simulink library "thc"  (R2021b)
settings: Solver=VariableStepAuto  StartTime=0.0  StopTime=10.0  RelTol=1e-3
undefined symbols (not defined in the file): ATHC_APTCQA_X_C, ATHC_APTCQB_X_C, ATHC_dAy_X_C, ATHC_Qeq_X_kmh, ATHC_VbaseC_X_C, ATHC_VbaseC_Y_W, ATHC_VbaseD_X_C, ATHC_VbaseH_X_C, FALSE, KTHC_ACMaxMinT_sec, KTHC_aDeice_K, KTHC_AGSDefLv_K, KTHC_AGSLv1_K, KTHC_AGSLv2_K, KTHC_AGSLv3_K, KTHC_AGSLv4_K, KTHC_AGSLv5_K, KTHC_AirIntUpdateT_sec, KTHC_APTCOneZoneMax_W, KTHC_APTCPeriod_cnt, KTHC_APTCPWMEN_flg, KTHC_APTCQMaxC_W, KTHC_APTCQminC_W, KTHC_APTCQminD_W, KTHC_APTCQminRe1_W, KTHC_APTCQminRe_W, KTHC_APTCQoffT_cnt, KTHC_APTCQonT_cnt, KTHC_APTCRiLeMaxDff_W, KTHC_APTCRiLeMinDff_W, KTHC_BatCoolT_cnt, KTHC_BatInTempDef_C, KTHC_bDeice_K, KTHC_CompMaxDeice_rpm, KTHC_CompMinDeice_rpm, KTHC_CompSotxvOp_K, KTHC_CompSotxvOpLow_rpm, KTHC_CompSpdmax_rpm, KTHC_CompSpdmaxBC1_rpm, KTHC_CompSpdmaxBC_rpm, KTHC_CompSpdmid1_rpm, KTHC_CompSpdmid2_rpm, KTHC_CompSpdmid3_rpm, KTHC_CompSpdmid_rpm, KTHC_CompSpdmin_rpm, KTHC_DAPTCQ1_W, KTHC_DAPTCQ2_W, KTHC_DAPTCQ3_W, KTHC_DcChSetTemp_C, KTHC_DehumidityEN_flg, KTHC_DeiceCycTime_K, KTHC_DriveLevelWPTCBAH1_W, KTHC_DriveLevelWPTCBAH2_W, KTHC_DriveLevelWPTCBAH3_W, KTHC_DriveLevelWPTCBAH4_W, KTHC_DriverSeatPos_flg, KTHC_DriveT1MinBAH_C, KTHC_DriveT2MaxBAH_C, KTHC_DriveT2MinBAH_C, KTHC_DriveT3MaxBAH_C ... (+379)
libraries: simulink x489
(part 1 of 17)
settings Model: Creator=FVT20341  LastModifiedBy=FVT22063

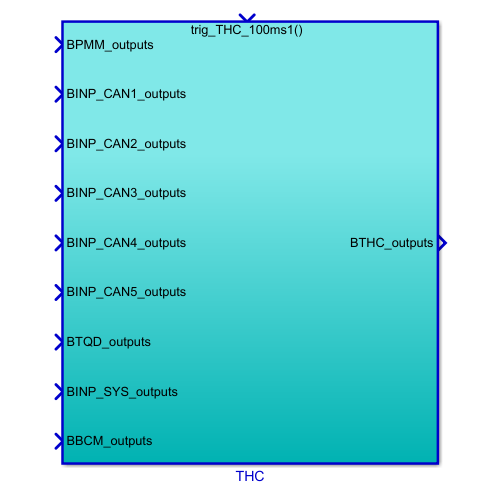
[thumbnail: Simulink's stored preview of the top-level diagram]
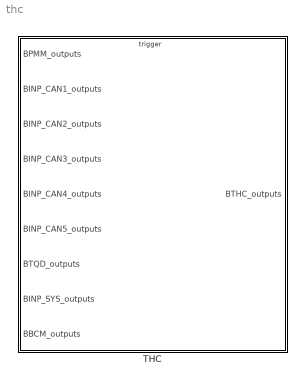
== system thc ==
  THC : Subsystem  TreatAsAtomicUnit=on
      settings: RTWSystemCode=Nonreusable function  RTWFcnNameOpts=Use subsystem name  RTWFileNameOpts=Use subsystem name

== system thc/THC ==
  BPMM_outputs : Inport  OutDataTypeStr=Bus: BPMM_outputs
  BINP_CAN1_outputs : Inport  Port=2  OutDataTypeStr=Bus: BINP_CAN1_outputs
  BINP_CAN2_outputs : Inport  Port=3  OutDataTypeStr=Bus: BINP_CAN2_outputs
  BINP_CAN3_outputs : Inport  Port=4  OutDataTypeStr=Bus: BINP_CAN3_outputs
  BINP_CAN4_outputs : Inport  Port=5  OutDataTypeStr=Bus: BINP_CAN4_outputs
  BINP_CAN5_outputs : Inport  Port=6  OutDataTypeStr=Bus: BINP_CAN5_outputs
  BTQD_outputs : Inport  Port=7  OutDataTypeStr=Bus: BTQD_outputs
  BINP_SYS_outputs : Inport  Port=8  OutDataTypeStr=Bus: BINP_SYS_outputs
  BBCM_outputs : Inport  Port=9  OutDataTypeStr=Bus: BBCM_outputs
  trig_THC_100ms1 : TriggerPort  TriggerType=function-call  VariantControl=(inherit)
  Bus Creator : BusCreator  Inputs=202  OutDataTypeStr=Bus: BTHC_outputs  NonVirtualBus=on
  Bus Selector : BusSelector  OutputSignals=VINP_FlashACModeMem_enum,VINP_FlashFace_enum,VINP_FlashFoot_enum,VINP_FlashFrost_enum,VINP_FlashFaceM_enum,VINP_FlashFootM_enum,VINP_FlashCCUSyncSts_enum,VINP_FlashACForceOFF_flg,VINP_FlashsigRecircSt_enum,VINP_FlashRecAutoFlg_enum,VINP_FlashAirIntenZone1M_enum,VINP_Flashfdefog_enum,VINP_FlashsigSetTempZon1St_C,VINP_FlashsigSetTempZon2StM_C,VINP_FlashAirIntZ3Sta_enum,VINP_FlashREVentModeSta_enum,VINP_FlashLEVentModeSta_enum,VINP_FlashLEVentZSta_enum,VINP_FlashCLEVentZSta_enum,VINP_FlashREVentZSta_enum,VINP_FlashCREVentZSta_enum,VINP_FlashLVentEN_enum,VINP_FlashLEVentYSta_enum,VINP_FlashCLVentEN_enum,VINP_FlashCLEVentYSta_enum,VINP_FlashRVentEN_enum,VINP_FlashREVentYSta_enum,VINP_FlashCRVentEN_enum,VINP_FlashCREVentYSta_enum,VINP_FlashFGSAirIntSta_enum,VINP_FlashFGSChSta_enum,VINP_FlashFGSIONSWSta_enum,VINP_FlashAirIntenZone1MSet2_enum,VINP_FlashAirIntenZone1MSet3_enum,VINP_FlashAirIntenZone1MSet4_enum,VINP_FlashAirIntenZone1MSet5_enum,VINP_FlashAirIntenZone1MSet7_enum,VINP_FlashAirIntenZone3MSet2_enum,VINP_FlashAirIntenZone3MSet3_enum,VINP_FlashAirIntenZone3MSet4_enum,VINP_FlashAirIntenZone3MSet5_enum,VINP_FlashAirIntenZone3MSet7_enum,VINP_FlashFGSChStaSet457_enum,VINP_FlashFGSAirIntStaSet457_enum,VINP_FlashLEVentModeStaSet457_enum,VINP_FlashREVentModeStaSet457_enum,VINP_FlashLEVentZStaSet2_enum,VINP_FlashLEVentZStaSet3_enum,VINP_FlashLEVentZStaSet4_enum,VINP_FlashLEVentZStaSet5_enum,VINP_FlashLEVentZStaSet7_enum,VINP_FlashCLEVentZStaSet2_enum,VINP_FlashCLEVentZStaSet3_enum,VINP_FlashCLEVentZStaSet4_enum,VINP_FlashCLEVentZStaSet5_enum,VINP_FlashCLEVentZStaSet7_enum,VINP_FlashREVentZStaSet2_enum,VINP_FlashREVentZStaSet3_enum,VINP_FlashREVentZStaSet4_enum,VINP_FlashREVentZStaSet5_enum,VINP_FlashREVentZStaSet7_enum,VINP_FlashCREVentZStaSet2_enum,VINP_FlashCREVentZStaSet3_enum,VINP_FlashCREVentZStaSet4_enum,VINP_FlashCREVentZStaSet5_enum,VINP_FlashCREVentZStaSet7_enum,VINP_FlashLEVentYStaSet2_enum,VINP_FlashLEVentYStaSet3_enum,VINP_FlashLEVentYStaSet4_enum,VINP_FlashLEVentYStaSet5_enum,VINP_FlashLEVentYStaSet7_enum,VINP_FlashCLEVentYStaSet2_enum,VINP_FlashCLEVentYStaSet3_enum,VINP_FlashCLEVentYStaSet4_enum,VINP_FlashCLEVentYStaSet5_enum,VINP_FlashCLEVentYStaSet7_enum,VINP_FlashREVentYStaSet2_enum,VINP_FlashREVentYStaSet3_enum,VINP_FlashREVentYStaSet4_enum,VINP_FlashREVentYStaSet5_enum,VINP_FlashREVentYStaSet7_enum,VINP_FlashCREVentYStaSet2_enum,VINP_FlashCREVentYStaSet3_enum,VINP_FlashCREVentYStaSet4_enum,VINP_FlashCREVentYStaSet5_enum,VINP_FlashCREVentYStaSet7_enum,VINP_FlashACModeSet457_enum,VINP_FlashSettempZon1Set2_enum,VINP_FlashSettempZon1Set3_enum,VINP_FlashSettempZon1Set4_enum,VINP_FlashSettempZon1Set5_enum,VINP_FlashSettempZon1Set7_enum
  Bus Selector1 : BusSelector  OutputSignals=VINP_VehSpeed_kph
  Bus Selector2 : BusSelector  OutputSignals=VINP_HVBMTempMax_C,VINP_HVBMTempMin_C,VINP_OBCTemp_C,VINP_DCDCTemp_C,VINP_RrTMTemp_C,VINP_RrMCUTemp_C,VINP_FrTMTemp_C,VINP_FrMCUTemp_C,VINP_ChrgPlugSta_enum,VINP_FrLLCTemp_C,VINP_RrLLCTemp_C,VINP_HVBIsoImpedenceN_Megaohm,VINP_HVBIsoImpedenceP_Megaohm,VINP_HVBHVILErr_flg,VINP_HVBattSOCDis_pct
  Bus Selector3 : BusSelector  OutputSignals=VINP_PTHighTact_C,VINP_COMPStatorSpd_rpm,VINP_CompProEN_flg,VINP_PTLowP1_KPa,VINP_PTLowT1_C,VINP_PTLowP2_KPa,VINP_PTLowT2_C,VINP_PTHighP_KPa,VINP_Tamb_C,VINP_BatInTemp_C,VINP_BatOutTemp_C,VINP_MotorInTemp_C,VINP_MotorOutTemp_C,VINP_Tincar_C,VINP_SolarL_W,VINP_SolarR_W,VINP_Tevap_C,VINP_TFaceL_C,VINP_TFaceR_C,VINP_TFootL_C,VINP_TFootR_C,VINP_TFootRr_C,VINP_TFaceRr_C,VINP_EACProtectEnable_enum,VINP_TambErr_enum,VINP_SolarLErr_enum,VINP_SolarRErr_enum,VINP_TevapErr_enum,VINP_TFaceLErr_enum,VINP_TFaceRErr_enum,VINP_TFootLErr_enum,VINP_TFootRErr_enum,VINP_TFaceRrErr_enum,VINP_TFootRrErr_enum,VINP_TincarErr_enum,VINP_BatInTempErr_enum,VINP_MotorInTempErr_enum,VINP_MotorOutTempErr_enum,VINP_FanErr_enum,VINP_AGSErr_enum,VINP_EWP3Err_enum,VINP_PTHighPErr_enum,VINP_PTHighTactErr_enum,VINP_SOV1Err_enum,VINP_SOV2Err_enum,VINP_SOV3Err_enum,VINP_EXV1Err_enum,VINP_EXV2Err_enum,VINP_COMPErr_enum,VINP_BlowerErr_enum,VINP_PTLowP1Err_enum,VINP_PTLowT1Err_enum,VINP_PTLowP2Err_enum,VINP_PTLowT2Err_enum,VINP_SOTXVErr_enum,VINP_FrntPTCRearLeActHeatPwr_W,VINP_FrntPTCRearRiActHeatPwr_W,VINP_FrntPTCRiActHeatPwr_W,VINP_ZFRTHCMLEVentActYSta_pct,VINP_ZFRTHCMCLEVentActYSta_pct,VINP_ZFRTHCMREVentActYSta_pct,VINP_ZFRTHCMCREVentActYSta_pct,VINP_FGSIntenRspSta_enum,VINP_EWP1BlockError_enum,VINP_EWP1OverCurrError_enum,VINP_EWP2BlockError_enum,VINP_EWP2OverCurrError_enum,VINP_EWP3BlockError_enum,VINP_EWP3OverCurrError_enum
  Bus Selector4 : BusSelector  OutputSignals=VINP_OFFACMODE_enum,VINP_FCPFrEvtBtnACMaxReq_flg,VINP_FCPFrEvtBtnACReq_flg,VINP_FCPFrEvtBtnAutoReq_flg,VINP_FCPFrEvtBtnSyncReq_flg,VINP_sigAirIntenZon1Req_enum,VINP_sigRecircReq_flg,VINP_sigFaceReq_flg,VINP_sigFootReq_flg,VINP_sigDfrstReq_flg,VINP_sigSetTempZon1Req_C,VINP_CANMsgValidIVI2_flg,VINP_sigSetTempZon2Req_C,VINP_SmartEcoModeSW_flg,VINP_HMIACBtnCmd_flg,VINP_HMIACAutoBtnCmd_flg,VINP_HMIACRecycleBtnCmd_flg,VINP_HMIACFrDefogBtnCmd_flg,VINP_HMIZLSetTPCmd_flg,VINP_HMIZLSetTMCmd_flg,VINP_HMIZRSetTPCmd_flg,VINP_HMIZRSetTMCmd_flg,VINP_HMIACWindDirPCmd_flg,VINP_HMIACWindDirMCmd_flg,VINP_HMIACAirIntPCmd_flg,VINP_HMIACAirIntMCmd_flg,VINP_IVIAirIntZ3Cmd_enum,VINP_IVILBlowerModeSta_enum,VINP_IVIRBlowerModeSta_enum,VINP_IVILBlowerZSta_pct,VINP_IVICLBlowerZSta_pct,VINP_IVIRBlowerZSta_pct,VINP_IVICRBlowerZSta_pct,VINP_IVILBlowerYSta_pct,VINP_IVICLBlowerYSta_pct,VINP_IVIRBlowerYSta_pct,VINP_IVICRBlowerYSta_pct,VINP_IVIsigScreenReqSta_flg,VINP_IVIFGSAirIntCmd_enum,VINP_IVIFGSChCmd_enum,VINP_IVIIONSWCmd_flg,VINP_IVIWPTCSWSta_flg,VINP_IVIZon1WindDirSWReqSta_flg
  Bus Selector5 : BusSelector  OutputSignals=VTQD_ShiftGearPosn_enum
  Bus Selector6 : BusSelector  OutputSignals=VINP_RemoteACTemp_C,VINP_RemoteAutoReq_flg
  Bus Selector7 : BusSelector  OutputSignals=VPMM_PowerSta_enum,VPMM_SysPowerMode_enum
  Bus Selector8 : BusSelector  OutputSignals=VBCM_UserNow_enum
  Ground{,1..3} (4 alike) : Ground
  Terminator : Terminator
  ThermalControl : Subsystem
  BTHC_outputs : Outport  OutDataTypeStr=Bus: BTHC_outputs
  wires:
  BPMM_outputs/1 -> Bus Selector7/1
  Bus Selector7/1 -> ThermalControl/1(VPMM_PwrSta_enum)  "<VPMM_PowerSta_enum>"
  BINP_CAN1_outputs/1 -> Bus Selector1/1
  Bus Selector1/1 -> ThermalControl/5(VINP_VehSpeed_kph)  "<VINP_VehSpeed_kph>"
  BINP_CAN3_outputs/1 -> Bus Selector2/1
  Bus Selector2/3 -> ThermalControl/8(VINP_OBCTemp_C)  "<VINP_OBCTemp_C>"
  Bus Selector2/4 -> ThermalControl/9(VINP_DCDCTemp_C)  "<VINP_DCDCTemp_C>"
  Bus Selector2/2 -> ThermalControl/7(VINP_HVBMTempMin_C)  "<VINP_HVBMTempMin_C>"
  Bus Selector2/5 -> ThermalControl/10(VINP_RrTMTemp_C)  "<VINP_RrTMTemp_C>"
  Bus Selector2/1 -> ThermalControl/6(VINP_HVBMTempMax_C)  "<VINP_HVBMTempMax_C>"
  Bus Selector2/6 -> ThermalControl/11(VINP_RrMCUTemp_C)  "<VINP_RrMCUTemp_C>"
  Bus Selector2/7 -> ThermalControl/12(VINP_FrTMTemp_C)  "<VINP_FrTMTemp_C>"
  Bus Selector2/8 -> ThermalControl/13(VINP_FrMCUTemp_C)  "<VINP_FrMCUTemp_C>"
  ThermalControl/32(VTHC_sigClntTHvBattOut_C) -> Bus Creator/32  "VTHC_sigClntTHvBattOut_C"
  ThermalControl/30(VTHC_sigSetTempZon1St_C) -> Bus Creator/30  "VTHC_sigSetTempZon1St_C"
  ThermalControl/29(VTHC_sigRecircSt_flg) -> Bus Creator/29  "VTHC_sigRecircSt_flg"
  ThermalControl/28(VTHC_sigWindDirZon1St_enum) -> Bus Creator/28  "VTHC_sigWindDirZon1St_enum"
  ThermalControl/27(VTHC_sigAirIntenZon1St_enum) -> Bus Creator/27  "VTHC_sigAirIntenZon1St_enum"
  ThermalControl/26(VTHC_CCUSyncLampSts_flg) -> Bus Creator/26  "VTHC_CCUSyncLampSts_flg"
  ThermalControl/25(VTHC_CCUACMaxLampSts_flg) -> Bus Creator/25  "VTHC_CCUACMaxLampSts_flg"
  ThermalControl/24(VTHC_CCUAutoLampSts_flg) -> Bus Creator/24  "VTHC_CCUAutoLampSts_flg"
  ThermalControl/23(VTHC_CCUACLampSts_flg) -> Bus Creator/23  "VTHC_CCUACLampSts_flg"
  ThermalControl/22(VTHC_CabinMode_enum) -> Bus Creator/22  "VTHC_CabinMode_enum"
  ThermalControl/21(VTHC_EDriveMode_enum) -> Bus Creator/21  "VTHC_EDriveMode_enum"
  ThermalControl/20(VTHC_BatteryMode_enum) -> Bus Creator/20  "VTHC_BatteryMode_enum"
  ThermalControl/19(VTHC_FDBlowerCmd_pct) -> Bus Creator/19  "VTHC_FDBlowerCmd_pct"
  ThermalControl/17(VTHC_FDFrRiAPTCHeatPwrCmd_W) -> Bus Creator/17  "VTHC_FDFrRiAPTCHeatPwrCmd_W"
  ThermalControl/18(VTHC_FDRrAPTCHeatPwrCmd_W) -> Bus Creator/18  "VTHC_FDRrAPTCHeatPwrCmd_W"
  ThermalControl/16(VTHC_FDFrLeAPTCHeatPwrCmd_W) -> Bus Creator/16  "VTHC_FDFrLeAPTCHeatPwrCmd_W"
  ThermalControl/15(VTHC_FDEWP3Cmd_enum) -> Bus Creator/15  "VTHC_FDEWP3Cmd_enum"
  ThermalControl/14(VTHC_FDEWP2Cmd_enum) -> Bus Creator/14  "VTHC_FDEWP2Cmd_enum"
  ThermalControl/13(VTHC_FDEWP1Cmd_enum) -> Bus Creator/13  "VTHC_FDEWP1Cmd_enum"
  ThermalControl/12(VTHC_FDAGSCmd_enum) -> Bus Creator/12  "VTHC_FDAGSCmd_enum"
  ThermalControl/11(VTHC_CoolgFanActDuty_pct) -> Bus Creator/11  "VTHC_CoolgFanActDuty_pct"
  ThermalControl/10(VTHC_FDFrWPTCHeatPwrCmd_W) -> Bus Creator/10  "VTHC_FDFrWPTCHeatPwrCmd_W"
  ThermalControl/9(VTHC_FDTWVCmd_pct) -> Bus Creator/9  "VTHC_FDTWVCmd_pct"
  ThermalControl/8(VTHC_FDFWVCmd_flg) -> Bus Creator/8  "VTHC_FDFWVCmd_flg"
  ThermalControl/7(VTHC_FDSOTXVCmd_flg) -> Bus Creator/7  "VTHC_FDSOTXVCmd_flg"
  ThermalControl/6(VTHC_FDEXV2Cmd_step) -> Bus Creator/6  "VTHC_FDEXV2Cmd_step"
  ThermalControl/5(VTHC_FDEXV1Cmd_step) -> Bus Creator/5  "VTHC_FDEXV1Cmd_step"
  ThermalControl/4(VTHC_FDSOV3Cmd_flg) -> Bus Creator/4  "VTHC_FDSOV3Cmd_flg"
  ThermalControl/3(VTHC_FDSOV2Cmd_flg) -> Bus Creator/3  "VTHC_FDSOV2Cmd_flg"
  ThermalControl/2(VTHC_FDSOV1Cmd_flg) -> Bus Creator/2  "VTHC_FDSOV1Cmd_flg"
  ThermalControl/1(VTHC_FDCompCmd_rpm) -> Bus Creator/1  "VTHC_FDCompCmd_rpm"
  Bus Creator/1 -> BTHC_outputs/1  "BTHC_outputs"
  BINP_CAN4_outputs/1 -> Bus Selector3/1  "BINP_CAN4_outputs"
  Bus Selector3/4 -> ThermalControl/24(VINP_PTLowP1_kPa)  "<VINP_PTLowP1_KPa>"
  Bus Selector3/5 -> ThermalControl/25(VINP_PTLowT1_C)  "<VINP_PTLowT1_C>"
  Bus Selector3/6 -> ThermalControl/26(VINP_PTLowP2_kPa)  "<VINP_PTLowP2_KPa>"
  Bus Selector3/7 -> ThermalControl/27(VINP_PTLowT2_C)  "<VINP_PTLowT2_C>"
  Bus Selector3/8 -> ThermalControl/28(VINP_PTHighP_kPa)  "<VINP_PTHighP_KPa>"
  Bus Selector3/9 -> ThermalControl/29(VINP_Tamb_C)  "<VINP_Tamb_C>"
  Bus Selector3/10 -> ThermalControl/30(VINP_BatInTemp_C)  "<VINP_BatInTemp_C>"
  Bus Selector3/11 -> ThermalControl/31(VINP_BatOutTemp_C)  "<VINP_BatOutTemp_C>"
  Bus Selector3/12 -> ThermalControl/32(VINP_MotorInTemp_C)  "<VINP_MotorInTemp_C>"
  Bus Selector3/13 -> ThermalControl/33(VINP_MotorOutTemp_C)  "<VINP_MotorOutTemp_C>"
  Bus Selector3/14 -> ThermalControl/34(VINP_Tincar_C)  "<VINP_Tincar_C>"
  Bus Selector3/15 -> ThermalControl/35(VINP_SolarL_W)  "<VINP_SolarL_W>"
  Bus Selector3/16 -> ThermalControl/36(VINP_SolarR_W)  "<VINP_SolarR_W>"
  Bus Selector3/17 -> ThermalControl/37(VINP_Tevap_C)  "<VINP_Tevap_C>"
  Bus Selector3/18 -> ThermalControl/38(VINP_TFaceL_C)  "<VINP_TFaceL_C>"
  Bus Selector3/19 -> ThermalControl/39(VINP_TFaceR_C)  "<VINP_TFaceR_C>"
  Bus Selector3/20 -> ThermalControl/40(VINP_TFootL_C)  "<VINP_TFootL_C>"
  Bus Selector3/21 -> ThermalControl/41(VINP_TFootR_C)  "<VINP_TFootR_C>"
  Bus Selector3/22 -> ThermalControl/42(VINP_TFootRr_C)  "<VINP_TFootRr_C>"
  Bus Selector3/23 -> ThermalControl/43(VINP_TFaceRr_C)  "<VINP_TFaceRr_C>"
  BINP_CAN2_outputs/1 -> Bus Selector4/1  "BINP_CAN2_outputs"
  Bus Selector4/2 -> ThermalControl/91(VINP_FCPFrEvtBtnACMaxReq_flg)  "<VINP_FCPFrEvtBtnACMaxReq_flg>"
  Bus Selector4/3 -> ThermalControl/92(VINP_FCPFrEvtBtnACReq_flg)  "<VINP_FCPFrEvtBtnACReq_flg>"
  Bus Selector4/4 -> ThermalControl/93(VINP_FCPFrEvtBtnAutoReq_flg)  "<VINP_FCPFrEvtBtnAutoReq_flg>"
  Bus Selector4/5 -> ThermalControl/94(VINP_FCPFrEvtBtnSyncReq_flg)  "<VINP_FCPFrEvtBtnSyncReq_flg>"
  Bus Selector4/6 -> ThermalControl/95(VINP_sigAirIntenZon1Req_enum)  "<VINP_sigAirIntenZon1Req_enum>"
  Bus Selector4/7 -> ThermalControl/96(VINP_sigRecircReq_flg)  "<VINP_sigRecircReq_flg>"
  Bus Selector4/8 -> ThermalControl/97(VINP_sigFaceReq_flg)  "<VINP_sigFaceReq_flg>"
  Bus Selector4/9 -> ThermalControl/98(VINP_sigFootReq_flg)  "<VINP_sigFootReq_flg>"
  Bus Selector4/10 -> ThermalControl/99(VINP_sigFrostReq_flg)  "<VINP_sigDfrstReq_flg>"
  Bus Selector4/11 -> ThermalControl/100(VINP_sigSetTempZon1Req_C)  "<VINP_sigSetTempZon1Req_C>"
  Bus Selector4/12 -> ThermalControl/101(VINP_CANMsgValidIVI2_flg)  "<VINP_CANMsgValidIVI2_flg>"
  Bus Selector4/13 -> ThermalControl/102(VINP_sigSetTempZon2Req_C)  "<VINP_sigSetTempZon2Req_C>"
  Bus Selector2/9 -> ThermalControl/14(VINP_ChrgPlugSta_enum)  "<VINP_ChrgPlugSta_enum>"
  Bus Selector3/2 -> ThermalControl/22(VINP_COMP_StatorSpd_RPM)  "<VINP_COMPStatorSpd_rpm>"
  Bus Selector3/3 -> ThermalControl/23(VINP_CompProEN_flg)  "<VINP_CompProEN_flg>"
  ThermalControl/33(VTHC_sigCbnSolarLeft_W) -> Bus Creator/33  "VTHC_sigCbnSolarLeft_W"
  ThermalControl/34(VTHC_sigClntTHvBattIn_C) -> Bus Creator/34  "VTHC_sigClntTHvBattIn_C"
  ThermalControl/35(VTHC_sigCbnSolarRight_W) -> Bus Creator/35  "VTHC_sigCbnSolarRight_W"
  ThermalControl/36(VTHC_sigAmbAirT_C) -> Bus Creator/36  "VTHC_sigAmbAirT_C"
  ThermalControl/37(VTHC_sigCbnAirT_C) -> Bus Creator/37  "VTHC_sigCbnAirT_C"
  ThermalControl/38(VTHC_ACSubMode_enum) -> Bus Creator/38  "VTHC_ACSubMode_enum"
  ThermalControl/40(VTHC_CompP_K) -> Bus Creator/40  "VTHC_CompP_K"
  ThermalControl/41(VTHC_CompI_K) -> Bus Creator/41  "VTHC_CompI_K"
  ThermalControl/42(VTHC_CompU_K) -> Bus Creator/42  "VTHC_CompU_K"
  ThermalControl/43(VTHC_CompDeltaU_K) -> Bus Creator/43  "VTHC_CompDeltaU_K"
  ThermalControl/44(VTHC_Compe_K) -> Bus Creator/44  "VTHC_Compe_K"
  ThermalControl/45(VTHC_Blowere_K) -> Bus Creator/45  "VTHC_Blowere_K"
  ThermalControl/46(VTHC_BlowerP_K) -> Bus Creator/46  "VTHC_BlowerP_K"
  ThermalControl/47(VTHC_BlowerU_K) -> Bus Creator/47  "VTHC_BlowerU_K"
  ThermalControl/48(VTHC_Vbase_pct) -> Bus Creator/48  "VTHC_Vbase_pct"
  ThermalControl/49(VTHC_BlowerI_K) -> Bus Creator/49  "VTHC_BlowerI_K"
  ThermalControl/50(VTHC_EXV2P_K) -> Bus Creator/50  "VTHC_EXV2P_K"
  ThermalControl/51(VTHC_EXV2I_K) -> Bus Creator/51  "VTHC_EXV2I_K"
  ThermalControl/52(VTHC_EXV2U_K) -> Bus Creator/52  "VTHC_EXV2U_K"
  ThermalControl/53(VTHC_EXV2e_K) -> Bus Creator/53  "VTHC_EXV2e_K"
  ThermalControl/54(VTHC_APTCP_K) -> Bus Creator/54  "VTHC_APTCP_K"
  ThermalControl/55(VTHC_APTCI_K) -> Bus Creator/55  "VTHC_APTCI_K"
  ThermalControl/56(VTHC_APTCU_K) -> Bus Creator/56  "VTHC_APTCU_K"
  ThermalControl/57(VTHC_APTCe_K) -> Bus Creator/57  "VTHC_APTCe_K"
  ThermalControl/58(VTHC_EXV1P_K) -> Bus Creator/58  "VTHC_EXV1P_K"
  ThermalControl/59(VTHC_EXV1I_K) -> Bus Creator/59  "VTHC_EXV1I_K"
  ThermalControl/60(VTHC_EXV1U_K) -> Bus Creator/60  "VTHC_EXV1U_K"
  ThermalControl/61(VTHC_EXV1e_K) -> Bus Creator/61  "VTHC_EXV1e_K"
  BTQD_outputs/1 -> Bus Selector5/1
  Bus Selector5/1 -> ThermalControl/3(VTQD_ShiftGearPosn_enum)  "<VTQD_ShiftGearPosn_enum>"
  Bus Selector3/1 -> ThermalControl/21(VINP_PTHighTact_C)  "<VINP_PTHighTact_C>"
  Bus Selector2/10 -> ThermalControl/15(VINP_FrLLCTemp_C)  "<VINP_FrLLCTemp_C>"
  Bus Selector2/11 -> ThermalControl/16(VINP_RrLLCTemp_C)  "<VINP_RrLLCTemp_C>"
  Ground/1 -> ThermalControl/4(VSCP_AGSCloseSta_flg)
  Bus Selector4/1 -> ThermalControl/90(VINP_OFFACMODE_enum)  "<VINP_OFFACMODE_enum>"
  ThermalControl/39(VTHC_FDRecyAutoCmd_enum) -> Bus Creator/39  "VTHC_FDRecyAutoCmd_enum"
  Bus Selector3/24 -> ThermalControl/44(VINP_EACProtectEnable_enum)  "<VINP_EACProtectEnable_enum>"
  Bus Selector3/25 -> ThermalControl/45(Tamb_Err)  "<VINP_TambErr_enum>"
  Bus Selector3/26 -> ThermalControl/46(SolarL_Err)  "<VINP_SolarLErr_enum>"
  Bus Selector3/27 -> ThermalControl/47(SolarR_Err)  "<VINP_SolarRErr_enum>"
  Bus Selector3/28 -> ThermalControl/48(Tevap_Err)  "<VINP_TevapErr_enum>"
  Bus Selector3/29 -> ThermalControl/49(T_Face_L_Err)  "<VINP_TFaceLErr_enum>"
  Bus Selector3/30 -> ThermalControl/50(T_Face_R_Err)  "<VINP_TFaceRErr_enum>"
  Bus Selector3/31 -> ThermalControl/51(T_Foot_L_Err)  "<VINP_TFootLErr_enum>"
  Bus Selector3/32 -> ThermalControl/52(T_Foot_R_Err)  "<VINP_TFootRErr_enum>"
  Bus Selector3/33 -> ThermalControl/53(T_Face_Rr_Err)  "<VINP_TFaceRrErr_enum>"
  Bus Selector3/34 -> ThermalControl/54(T_Foot_Rr_Err)  "<VINP_TFootRrErr_enum>"
  Bus Selector3/35 -> ThermalControl/55(Tincar_Err)  "<VINP_TincarErr_enum>"
  Bus Selector3/36 -> ThermalControl/56(Bat_In_Temp_Err)  "<VINP_BatInTempErr_enum>"
  Bus Selector3/37 -> ThermalControl/57(Motor_In_Temp_Err)  "<VINP_MotorInTempErr_enum>"
  Bus Selector3/38 -> ThermalControl/58(Motor_Out_Temp_Err)  "<VINP_MotorOutTempErr_enum>"
  Bus Selector3/39 -> ThermalControl/59(Fan_Err)  "<VINP_FanErr_enum>"
  Bus Selector3/40 -> ThermalControl/60(AGS_Err)  "<VINP_AGSErr_enum>"
  Bus Selector3/41 -> ThermalControl/61(EWP3_Err)  "<VINP_EWP3Err_enum>"
  Bus Selector3/42 -> ThermalControl/62(PT_High_P_Err)  "<VINP_PTHighPErr_enum>"
  Bus Selector3/43 -> ThermalControl/63(PT_High_Tact_Err)  "<VINP_PTHighTactErr_enum>"
  Bus Selector3/44 -> ThermalControl/64(SOV1_Err)  "<VINP_SOV1Err_enum>"
  Bus Selector3/45 -> ThermalControl/65(SOV2_Err)  "<VINP_SOV2Err_enum>"
  Bus Selector3/46 -> ThermalControl/66(SOV3_Err)  "<VINP_SOV3Err_enum>"
  Bus Selector3/47 -> ThermalControl/67(EXV1_Err)  "<VINP_EXV1Err_enum>"
  Bus Selector3/48 -> ThermalControl/68(EXV2_Err)  "<VINP_EXV2Err_enum>"
  Bus Selector3/49 -> ThermalControl/69(Comp_Err)  "<VINP_COMPErr_enum>"
  Bus Selector3/50 -> ThermalControl/70(Blower_Err)  "<VINP_BlowerErr_enum>"
  Bus Selector3/51 -> ThermalControl/71(PT_Low_P1_Err)  "<VINP_PTLowP1Err_enum>"
  Bus Selector3/52 -> ThermalControl/72(PT_Low_T1_Err)  "<VINP_PTLowT1Err_enum>"
  Bus Selector3/53 -> ThermalControl/73(PT_Low_P2_Err)  "<VINP_PTLowP2Err_enum>"
  Bus Selector3/54 -> ThermalControl/74(PT_Low_T2_Err)  "<VINP_PTLowT2Err_enum>"
  Bus Selector3/55 -> ThermalControl/75(SOTXV_Err)  "<VINP_SOTXVErr_enum>"
  ThermalControl/62(VTHC_ACModeMem_enum) -> Bus Creator/62  "VTHC_ACModeMem_enum"
  ThermalControl/63(VTHC_Face_flg) -> Bus Creator/63  "VTHC_Face_flg"
  ThermalControl/64(VTHC_Foot_flg) -> Bus Creator/64  "VTHC_Foot_flg"
  ThermalControl/65(VTHC_Frost_flg) -> Bus Creator/65  "VTHC_Frost_flg"
  ThermalControl/66(VTHC_FaceM_flg) -> Bus Creator/66  "VTHC_FaceM_flg"
  ThermalControl/67(VTHC_FootM_flg) -> Bus Creator/67  "VTHC_FootM_flg"
  ThermalControl/68(VTHC_CCUSyncSts_flg) -> Bus Creator/68  "VTHC_CCUSyncSts_flg"
  ThermalControl/69(VTHC_ACForceOFF_flg) -> Bus Creator/69  "VTHC_ACForceOFF_flg"
  ThermalControl/70(VTHC_RecAutoFlg_flg) -> Bus Creator/70  "VTHC_RecAutoFlg_flg"
  ThermalControl/71(VTHC_AirIntenZone1M_enum) -> Bus Creator/71  "VTHC_AirIntenZone1M_enum"
  ThermalControl/72(VTHC_fdefog_flg) -> Bus Creator/72  "VTHC_fdefog_flg"
  Bus Selector/8 -> ThermalControl/143(EEP_ACForceOFF)  "<VINP_FlashACForceOFF_flg>"
  Bus Selector/10 -> ThermalControl/145(EEP_RecyAutoSet)  "<VINP_FlashRecAutoFlg_enum>"
  ThermalControl/73(VTHC_sigSetTempZon2StM_C) -> Bus Creator/73
  Ground1/1 -> ThermalControl/133(ECOSW)
  Bus Selector6/2 -> ThermalControl/135(VINP_RemoteAutoReq_flg)  "<VINP_RemoteAutoReq_flg>"
  Bus Selector6/1 -> ThermalControl/134(VINP_RemoteACTemp_C)  "<VINP_RemoteACTemp_C>"
  Bus Selector4/14 -> ThermalControl/103(VINP_SmartEcoModeSW_flg)  "<VINP_SmartEcoModeSW_flg>"
  Bus Selector2/12 -> ThermalControl/17(VINP_HVBIsoImpedenceN_Mohm)  "<VINP_HVBIsoImpedenceN_Megaohm>"
  Bus Selector2/13 -> ThermalControl/18(VINP_HVBIsoImpedenceP_Mohm)  "<VINP_HVBIsoImpedenceP_Megaohm>"
  Bus Selector2/14 -> ThermalControl/19(VINP_HVBHVILErr_flg)  "<VINP_HVBHVILErr_flg>"
  Bus Selector3/56 -> ThermalControl/76(VINP_FrntPTCRearLeActHeatPwr_W)  "<VINP_FrntPTCRearLeActHeatPwr_W>"
  Bus Selector3/57 -> ThermalControl/77(VINP_FrntPTCRearRiActHeatPwr_W)  "<VINP_FrntPTCRearRiActHeatPwr_W>"
  Bus Selector3/58 -> ThermalControl/78(VINP_FrntPTCRiActHeatPwr_W)  "<VINP_FrntPTCRiActHeatPwr_W>"
  ThermalControl/74(VTHC_sigDfrstSt_flg) -> Bus Creator/74
  ThermalControl/75(VTHC_FDCTHCAirIntZ3Sta_enum) -> Bus Creator/75
  ThermalControl/76(VTHC_FDCTHCLEVentModeSta_enum) -> Bus Creator/76
  ThermalControl/77(VTHC_FDCTHCREVentModeSta_enum) -> Bus Creator/77
  ThermalControl/78(VTHC_FDCTHCLEVentZSta_enum) -> Bus Creator/78
  ThermalControl/79(VTHC_FDCTHCCLEVentZSta_enum) -> Bus Creator/79
  ThermalControl/80(VTHC_FDCTHCREVentZSta_enum) -> Bus Creator/80
  ThermalControl/81(VTHC_FDCTHCCREVentZSta_enum) -> Bus Creator/81
  ThermalControl/82(VTHC_FDCTHCLEVentYSta_enum) -> Bus Creator/82
  ThermalControl/83(VTHC_FDCTHCLVentENSta_flg) -> Bus Creator/83
  ThermalControl/84(VTHC_FDCTHCCLEVentYSta_enum) -> Bus Creator/84
  ThermalControl/85(VTHC_FDCTHCCLVentENSta_flg) -> Bus Creator/85
  ThermalControl/86(VTHC_FDCTHCREVentYSta_enum) -> Bus Creator/86
  ThermalControl/87(VTHC_FDCTHCRVentENSta_flg) -> Bus Creator/87
  ThermalControl/88(VTHC_FDCTHCCREVentYSta_enum) -> Bus Creator/88
  ThermalControl/89(VTHC_FDCTHCCRVentENSta_flg) -> Bus Creator/89
  ThermalControl/90(VTHC_FDCTHCMAPTCForceOFFSta_flg) -> Bus Creator/90
  Bus Selector/29 -> ThermalControl/164(EEP_FDCTHCCREVentYStaSet1)  "<VINP_FlashCREVentYSta_enum>"
  Bus Selector/31 -> ThermalControl/166(EEP_FDCFGSChStaSet123)  "<VINP_FlashFGSChSta_enum>"
  Bus Selector/30 -> ThermalControl/165(EEP_FDCFGSAirIntStaSet123)  "<VINP_FlashFGSAirIntSta_enum>"
  Bus Selector2/15 -> ThermalControl/20(VINP_HVBattSOC_pct)  "<VINP_HVBattSOCDis_pct>"
  Bus Selector3/59 -> ThermalControl/79(VINP_ZFRTHCLEVentActYSta_enum)  "<VINP_ZFRTHCMLEVentActYSta_pct>"
  Bus Selector3/60 -> ThermalControl/80(VINP_ZFRTHCCLEVentActYSta_enum)  "<VINP_ZFRTHCMCLEVentActYSta_pct>"
  Bus Selector3/61 -> ThermalControl/81(VINP_ZFRTHCREVentActYSta_enum)  "<VINP_ZFRTHCMREVentActYSta_pct>"
  Bus Selector3/62 -> ThermalControl/82(VINP_ZFRTHCCREVentActYSta_enum)  "<VINP_ZFRTHCMCREVentActYSta_pct>"
  Bus Selector4/15 -> ThermalControl/104(VINP_HMIACBtnCmd_flg)  "<VINP_HMIACBtnCmd_flg>"
  Bus Selector4/16 -> ThermalControl/105(VINP_HMIACAutoBtnCmd_flg)  "<VINP_HMIACAutoBtnCmd_flg>"
  Bus Selector4/17 -> ThermalControl/106(VINP_HMIACRecycleBtnCmd_flg)  "<VINP_HMIACRecycleBtnCmd_flg>"
  Bus Selector4/18 -> ThermalControl/107(VINP_HMIACFrDefogBtnCmd_flg)  "<VINP_HMIACFrDefogBtnCmd_flg>"
  Bus Selector4/19 -> ThermalControl/108(VINP_HMIZLSetTPCmd_flg)  "<VINP_HMIZLSetTPCmd_flg>"
  Bus Selector4/20 -> ThermalControl/109(VINP_HMIZLSetTMCmd_flg)  "<VINP_HMIZLSetTMCmd_flg>"
  Bus Selector4/21 -> ThermalControl/110(VINP_HMIZRSetTPCmd_flg)  "<VINP_HMIZRSetTPCmd_flg>"
  Bus Selector4/22 -> ThermalControl/111(VINP_HMIZRSetTMCmd_flg)  "<VINP_HMIZRSetTMCmd_flg>"
  Bus Selector4/23 -> ThermalControl/112(VINP_HMIACWindDirPCmd_flg)  "<VINP_HMIACWindDirPCmd_flg>"
  Bus Selector4/24 -> ThermalControl/113(VINP_HMIACWindDirMCmd_flg)  "<VINP_HMIACWindDirMCmd_flg>"
  Bus Selector4/25 -> ThermalControl/114(VINP_HMIACAirIntPCmd_flg)  "<VINP_HMIACAirIntPCmd_flg>"
  Bus Selector4/26 -> ThermalControl/115(VINP_HMIACAirIntMCmd_flg)  "<VINP_HMIACAirIntMCmd_flg>"
  Bus Selector4/27 -> ThermalControl/116(VINP_IVIAirIntZ3Cmd_enum)  "<VINP_IVIAirIntZ3Cmd_enum>"
  Bus Selector4/28 -> ThermalControl/117(VINP_IVILBlowerModeSta_enum)  "<VINP_IVILBlowerModeSta_enum>"
  Bus Selector4/29 -> ThermalControl/118(VINP_IVIRBlowerModeSta_enum)  "<VINP_IVIRBlowerModeSta_enum>"
  Bus Selector4/30 -> ThermalControl/119(VINP_IVILBlowerZSta_enum)  "<VINP_IVILBlowerZSta_pct>"
  Bus Selector4/31 -> ThermalControl/120(VINP_IVICLBlowerZSta_enum)  "<VINP_IVICLBlowerZSta_pct>"
  Bus Selector4/32 -> ThermalControl/121(VINP_IVIRBlowerZSta_enum)  "<VINP_IVIRBlowerZSta_pct>"
  Bus Selector4/33 -> ThermalControl/122(VINP_IVICRBlowerZSta_enum)  "<VINP_IVICRBlowerZSta_pct>"
  Bus Selector4/34 -> ThermalControl/123(VINP_IVILBlowerYSta_enum)  "<VINP_IVILBlowerYSta_pct>"
  Bus Selector4/35 -> ThermalControl/124(VINP_IVICLBlowerYSta_enum)  "<VINP_IVICLBlowerYSta_pct>"
  Bus Selector4/36 -> ThermalControl/125(VINP_IVIRBlowerYSta_enum)  "<VINP_IVIRBlowerYSta_pct>"
  Bus Selector4/37 -> ThermalControl/126(VINP_IVICRBlowerYSta_enum)  "<VINP_IVICRBlowerYSta_pct>"
  Bus Selector4/38 -> ThermalControl/127(VINP_IVIsigScreenReq_Sta)  "<VINP_IVIsigScreenReqSta_flg>"
  Bus Selector4/39 -> ThermalControl/128(VINP_IVIFGSAirIntCmd_enum)  "<VINP_IVIFGSAirIntCmd_enum>"
  Bus Selector4/40 -> ThermalControl/129(VINP_IVIFGSChCmd_enum)  "<VINP_IVIFGSChCmd_enum>"
  Bus Selector4/41 -> ThermalControl/130(VINP_IVIIONSWCmd_flg)  "<VINP_IVIIONSWCmd_flg>"
  Bus Selector4/42 -> ThermalControl/131(VINP_IVIWPTCSWSta_flg)  "<VINP_IVIWPTCSWSta_flg>"
  Bus Selector4/43 -> ThermalControl/132(VINP_IVIZon1WindDirSWReqSta_flg)  "<VINP_IVIZon1WindDirSWReqSta_flg>"
  Bus Selector/1 -> ThermalControl/136(EEP_ACModeSet123)  "<VINP_FlashACModeMem_enum>"
  Bus Selector/9 -> ThermalControl/144(EEP_sigRecircStSet)  "<VINP_FlashsigRecircSt_enum>"
  Bus Selector/11 -> ThermalControl/146(EEP_AirIntenZone1MSet1)  "<VINP_FlashAirIntenZone1M_enum>"
  Bus Selector/12 -> ThermalControl/147(EEP_fdefogSet)  "<VINP_Flashfdefog_enum>"
  Bus Selector/15 -> ThermalControl/150(EEP_AirIntenZone3MSet1)  "<VINP_FlashAirIntZ3Sta_enum>"
  Bus Selector/16 -> ThermalControl/151(EEP_FDCTHCREVentModeStaSet123)  "<VINP_FlashREVentModeSta_enum>"
  Bus Selector/17 -> ThermalControl/152(EEP_FDCTHCLEVentModeStaSet123)  "<VINP_FlashLEVentModeSta_enum>"
  Bus Selector/18 -> ThermalControl/153(EEP_FDCTHCLEVentZStaSet1)  "<VINP_FlashLEVentZSta_enum>"
  Bus Selector/19 -> ThermalControl/154(EEP_FDCTHCCLEVentZStaSet1)  "<VINP_FlashCLEVentZSta_enum>"
  Bus Selector/20 -> ThermalControl/155(EEP_FDCTHCREVentZStaSet1)  "<VINP_FlashREVentZSta_enum>"
  Bus Selector/21 -> ThermalControl/156(EEP_FDCTHCCREVentZStaSet1)  "<VINP_FlashCREVentZSta_enum>"
  Bus Selector/22 -> ThermalControl/157(EEP_LVentENSet)  "<VINP_FlashLVentEN_enum>"
  Bus Selector/23 -> ThermalControl/158(EEP_FDCTHCLEVentYStaSet1)  "<VINP_FlashLEVentYSta_enum>"
  Bus Selector/24 -> ThermalControl/159(EEP_CLVentENSet)  "<VINP_FlashCLVentEN_enum>"
  Bus Selector/25 -> ThermalControl/160(EEP_FDCTHCCLEVentYStaSet1)  "<VINP_FlashCLEVentYSta_enum>"
  Bus Selector/26 -> ThermalControl/161(EEP_RVentENSet)  "<VINP_FlashRVentEN_enum>"
  Bus Selector/27 -> ThermalControl/162(EEP_FDCTHCREVentYStaSet1)  "<VINP_FlashREVentYSta_enum>"
  Bus Selector/28 -> ThermalControl/163(EEP_CRVentENSet)  "<VINP_FlashCRVentEN_enum>"
  Bus Selector/14 -> ThermalControl/149(EEP_sigSetTempZon2StM)  "<VINP_FlashsigSetTempZon2StM_C>"
  ThermalControl/91(VTHC_Z1TUP_flg) -> Bus Creator/91
  ThermalControl/92(VTHC_Z1TDN_flg) -> Bus Creator/92
  ThermalControl/93(VTHC_Z2TUP_flg) -> Bus Creator/93
  ThermalControl/94(VTHC_Z2TDN_flg) -> Bus Creator/94
  ThermalControl/95(VTHC_FDCFGSAirIntSta_enum) -> Bus Creator/95
  ThermalControl/96(VTHC_FDCFGSChSta_enum) -> Bus Creator/96
  ThermalControl/97(VTHC_FDCFGSAirIntCmd_enum) -> Bus Creator/97
  ThermalControl/98(VTHC_FDCFGSFuncSta_enum) -> Bus Creator/98
  ThermalControl/99(VTHC_FDCFGSChCmd_enum) -> Bus Creator/99
  ThermalControl/100(VTHC_FDCFGSIONSWSta_flg) -> Bus Creator/100
  ThermalControl/101(VTHC_FDCFGSIONCmd_flg) -> Bus Creator/101
  ThermalControl/102(VTHC_FDCTHCMPreWPTCHeatSta_enum) -> Bus Creator/102
  ThermalControl/103(VTHC_EWPBUflag1_flg) -> Bus Creator/103
  ThermalControl/104(VTHC_EWPBUflag2_flg) -> Bus Creator/104
  ThermalControl/105(VTHC_EWPBUflag3_flg) -> Bus Creator/105
  ThermalControl/106(VTHC_FaceMSet_enum) -> Bus Creator/106
  ThermalControl/107(VTHC_FootMSet_enum) -> Bus Creator/107
  ThermalControl/108(VTHC_fdefogSet_enum) -> Bus Creator/108
  ThermalControl/109(VTHC_CCUSyncStsSet_enum) -> Bus Creator/109
  ThermalControl/110(VTHC_sigRecircStSet_enum) -> Bus Creator/110
  ThermalControl/111(VTHC_RecyAutoSet_enum) -> Bus Creator/111
  ThermalControl/112(VTHC_AirIntenZone1MSet1_enum) -> Bus Creator/112
  ThermalControl/113(VTHC_AirIntenZone1MSet2_enum) -> Bus Creator/113
  ThermalControl/114(VTHC_AirIntenZone1MSet3_enum) -> Bus Creator/114
  ThermalControl/115(VTHC_AirIntenZone1MSet4_enum) -> Bus Creator/115
  ThermalControl/116(VTHC_AirIntenZone1MSet5_enum) -> Bus Creator/116
  ThermalControl/117(VTHC_AirIntenZone1MSet7_enum) -> Bus Creator/117
  ThermalControl/118(VTHC_AirIntenZone3MSet1_enum) -> Bus Creator/118
  ThermalControl/119(VTHC_AirIntenZone3MSet2_enum) -> Bus Creator/119
  ThermalControl/120(VTHC_AirIntenZone3MSet3_enum) -> Bus Creator/120
  ThermalControl/121(VTHC_AirIntenZone3MSet4_enum) -> Bus Creator/121
  ThermalControl/122(VTHC_AirIntenZone3MSet5_enum) -> Bus Creator/122
  ThermalControl/123(VTHC_AirIntenZone3MSet7_enum) -> Bus Creator/123
  ThermalControl/124(VTHC_IONSWStaSet_enum) -> Bus Creator/124
  ThermalControl/125(VTHC_FDCFGSChStaSet123_enum) -> Bus Creator/125
  ThermalControl/126(VTHC_FDCFGSChStaSet457_enum) -> Bus Creator/126
  ThermalControl/127(VTHC_FDCFGSAirIntStaSet123_enum) -> Bus Creator/127
  ThermalControl/128(VTHC_FDCFGSAirIntStaSet457_enum) -> Bus Creator/128
  ThermalControl/129(VTHC_LVentENSet_enum) -> Bus Creator/129
  ThermalControl/130(VTHC_CLVentENSet_enum) -> Bus Creator/130
  ThermalControl/131(VTHC_RVentENSet_enum) -> Bus Creator/131
  ThermalControl/132(VTHC_CRVentENSet_enum) -> Bus Creator/132
  ThermalControl/133(VTHC_LEVentModeStaSet123_enum) -> Bus Creator/133
  ThermalControl/134(VTHC_LEVentModeStaSet457_enum) -> Bus Creator/134
  ThermalControl/135(VTHC_REVentModeStaSet123_enum) -> Bus Creator/135
  ThermalControl/136(VTHC_REVentModeStaSet457_enum) -> Bus Creator/136
  ThermalControl/137(VTHC_FDCTHCLEVentZStaSet1_enum) -> Bus Creator/137
  ThermalControl/138(VTHC_FDCTHCLEVentZStaSet2_enum) -> Bus Creator/138
  ThermalControl/139(VTHC_FDCTHCLEVentZStaSet3_enum) -> Bus Creator/139
  ThermalControl/140(VTHC_FDCTHCLEVentZStaSet4_enum) -> Bus Creator/140
  ThermalControl/141(VTHC_FDCTHCLEVentZStaSet5_enum) -> Bus Creator/141
  ThermalControl/142(VTHC_FDCTHCLEVentZStaSet7_enum) -> Bus Creator/142
  ThermalControl/143(VTHC_FDCTHCCLEVentZStaSet1_enum) -> Bus Creator/143
  ThermalControl/144(VTHC_FDCTHCCLEVentZStaSet2_enum) -> Bus Creator/144
  ThermalControl/145(VTHC_FDCTHCCLEVentZStaSet3_enum) -> Bus Creator/145
  ThermalControl/146(VTHC_FDCTHCCLEVentZStaSet4_enum) -> Bus Creator/146
  ThermalControl/147(VTHC_FDCTHCCLEVentZStaSet5_enum) -> Bus Creator/147
  ThermalControl/148(VTHC_FDCTHCCLEVentZStaSet7_enum) -> Bus Creator/148
  ThermalControl/149(VTHC_FDCTHCREVentZStaSet1_enum) -> Bus Creator/149
  ThermalControl/150(VTHC_FDCTHCREVentZStaSet2_enum) -> Bus Creator/150
  ThermalControl/151(VTHC_FDCTHCREVentZStaSet3_enum) -> Bus Creator/151
  ThermalControl/152(VTHC_FDCTHCREVentZStaSet4_enum) -> Bus Creator/152
  ThermalControl/153(VTHC_FDCTHCREVentZStaSet5_enum) -> Bus Creator/153
  ThermalControl/154(VTHC_FDCTHCREVentZStaSet7_enum) -> Bus Creator/154
  ThermalControl/155(VTHC_FDCTHCCREVentZStaSet1_enum) -> Bus Creator/155
  ThermalControl/156(VTHC_FDCTHCCREVentZStaSet2_enum) -> Bus Creator/156
  ThermalControl/157(VTHC_FDCTHCCREVentZStaSet3_enum) -> Bus Creator/157
  ThermalControl/158(VTHC_FDCTHCCREVentZStaSet4_enum) -> Bus Creator/158
  ThermalControl/159(VTHC_FDCTHCCREVentZStaSet5_enum) -> Bus Creator/159
  ThermalControl/160(VTHC_FDCTHCCREVentZStaSet7_enum) -> Bus Creator/160
  ThermalControl/161(VTHC_FDCTHCLEVentYStaSet1_enum) -> Bus Creator/161
  ThermalControl/162(VTHC_FDCTHCLEVentYStaSet2_enum) -> Bus Creator/162
  ThermalControl/163(VTHC_FDCTHCLEVentYStaSet3_enum) -> Bus Creator/163
  ThermalControl/164(VTHC_FDCTHCLEVentYStaSet4_enum) -> Bus Creator/164
  ThermalControl/165(VTHC_FDCTHCLEVentYStaSet5_enum) -> Bus Creator/165
  ThermalControl/166(VTHC_FDCTHCLEVentYStaSet7_enum) -> Bus Creator/166
  ThermalControl/167(VTHC_FDCTHCCLEVentYStaSet1_enum) -> Bus Creator/167
  ThermalControl/168(VTHC_FDCTHCCLEVentYStaSet2_enum) -> Bus Creator/168
  ThermalControl/169(VTHC_FDCTHCCLEVentYStaSet3_enum) -> Bus Creator/169
  ThermalControl/170(VTHC_FDCTHCCLEVentYStaSet4_enum) -> Bus Creator/170
  ThermalControl/171(VTHC_FDCTHCCLEVentYStaSet5_enum) -> Bus Creator/171
  ThermalControl/172(VTHC_FDCTHCCLEVentYStaSet7_enum) -> Bus Creator/172
  ThermalControl/173(VTHC_FDCTHCREVentYStaSet1_enum) -> Bus Creator/173
  ThermalControl/174(VTHC_FDCTHCREVentYStaSet2_enum) -> Bus Creator/174
  ThermalControl/175(VTHC_FDCTHCREVentYStaSet3_enum) -> Bus Creator/175
  ThermalControl/176(VTHC_FDCTHCREVentYStaSet4_enum) -> Bus Creator/176
  ThermalControl/177(VTHC_FDCTHCREVentYStaSet5_enum) -> Bus Creator/177
  ThermalControl/178(VTHC_FDCTHCREVentYStaSet7_enum) -> Bus Creator/178
  ThermalControl/179(VTHC_FDCTHCCREVentYStaSet1_enum) -> Bus Creator/179
  ThermalControl/180(VTHC_FDCTHCCREVentYStaSet2_enum) -> Bus Creator/180
  ThermalControl/181(VTHC_FDCTHCCREVentYStaSet3_enum) -> Bus Creator/181
  ThermalControl/182(VTHC_FDCTHCCREVentYStaSet4_enum) -> Bus Creator/182
  ThermalControl/183(VTHC_FDCTHCCREVentYStaSet5_enum) -> Bus Creator/183
  ThermalControl/184(VTHC_FDCTHCCREVentYStaSet7_enum) -> Bus Creator/184
  ThermalControl/185(VTHC_SettempZon1Set1_enum) -> Bus Creator/185
  ThermalControl/186(VTHC_SettempZon1Set2_enum) -> Bus Creator/186
  ThermalControl/187(VTHC_SettempZon1Set3_enum) -> Bus Creator/187
  ThermalControl/188(VTHC_SettempZon1Set4_enum) -> Bus Creator/188
  ThermalControl/189(VTHC_SettempZon1Set5_enum) -> Bus Creator/189
  ThermalControl/190(VTHC_SettempZon1Set7_enum) -> Bus Creator/190
  ThermalControl/191(VTHC_ACModeSet123_enum) -> Bus Creator/191
  ThermalControl/192(VTHC_ACModeSet457_enum) -> Bus Creator/192
  ThermalControl/193(VTHC_FACESet_enum) -> Bus Creator/193
  ThermalControl/194(VTHC_FOOTSet_enum) -> Bus Creator/194
  ThermalControl/195(VTHC_FrostSet_enum) -> Bus Creator/195
  Bus Selector3/63 -> ThermalControl/83(VINP_FGSAirIntSta_enum)  "<VINP_FGSIntenRspSta_enum>"
  Bus Selector3/64 -> ThermalControl/84("VINP_EWP1BlockError_enum ")  "<VINP_EWP1BlockError_enum>"
  Bus Selector3/65 -> ThermalControl/85(VINP_EWP1OverCurrError_enum)  "<VINP_EWP1OverCurrError_enum>"
  Bus Selector3/66 -> ThermalControl/86(VINP_EWP2BlockError_enum)  "<VINP_EWP2BlockError_enum>"
  Bus Selector3/67 -> ThermalControl/87(VINP_EWP2OverCurrError_enum)  "<VINP_EWP2OverCurrError_enum>"
  Bus Selector3/68 -> ThermalControl/88(VINP_EWP3BlockError_enum)  "<VINP_EWP3BlockError_enum>"
  Bus Selector3/69 -> ThermalControl/89(VINP_EWP3OverCurrError_enum)  "<VINP_EWP3OverCurrError_enum>"
  BBCM_outputs/1 -> Bus Selector8/1  "BBCM_outputs"
  Bus Selector8/1 -> ThermalControl/228(VBCM_UserNow_enum)  "<VBCM_UserNow_enum>"
  ThermalControl/31(VTHC_sigSetTempZon2St_C) -> Bus Creator/31  "VTHC_sigSetTempZon2St_C"
  Ground2/1 -> ThermalControl/229(VINP_UpdateReq_enum)
  Ground3/1 -> ThermalControl/230(APTCFailDTC)
  Bus Selector/2 -> ThermalControl/137(EEP_FACESet)  "<VINP_FlashFace_enum>"
  Bus Selector/3 -> ThermalControl/138(EEP_FOOTSet)  "<VINP_FlashFoot_enum>"
  Bus Selector/4 -> ThermalControl/139(EEP_FrostSet)  "<VINP_FlashFrost_enum>"
  Bus Selector/5 -> ThermalControl/140(EEP_FaceMSet)  "<VINP_FlashFaceM_enum>"
  Bus Selector/6 -> ThermalControl/141(EEP_FootMSet)  "<VINP_FlashFootM_enum>"
  Bus Selector/7 -> ThermalControl/142(EEP_CCUSyncStsSet)  "<VINP_FlashCCUSyncSts_enum>"
  Bus Selector/32 -> ThermalControl/167(EEP_IONSWStaSet)  "<VINP_FlashFGSIONSWSta_enum>"
  Bus Selector/33 -> ThermalControl/168(EEP_AirIntenZone1MSet2)  "<VINP_FlashAirIntenZone1MSet2_enum>"
  Bus Selector/34 -> ThermalControl/169(EEP_AirIntenZone1MSet3)  "<VINP_FlashAirIntenZone1MSet3_enum>"
  Bus Selector/35 -> ThermalControl/170(EEP_AirIntenZone1MSet4)  "<VINP_FlashAirIntenZone1MSet4_enum>"
  Bus Selector/36 -> ThermalControl/171(EEP_AirIntenZone1MSet5)  "<VINP_FlashAirIntenZone1MSet5_enum>"
  Bus Selector/37 -> ThermalControl/172(EEP_AirIntenZone1MSet7)  "<VINP_FlashAirIntenZone1MSet7_enum>"
  Bus Selector/38 -> ThermalControl/173(EEP_AirIntenZone3MSet2)  "<VINP_FlashAirIntenZone3MSet2_enum>"
  Bus Selector/39 -> ThermalControl/174(EEP_AirIntenZone3MSet3)  "<VINP_FlashAirIntenZone3MSet3_enum>"
  Bus Selector/40 -> ThermalControl/175(EEP_AirIntenZone3MSet4)  "<VINP_FlashAirIntenZone3MSet4_enum>"
  Bus Selector/41 -> ThermalControl/176(EEP_AirIntenZone3MSet5)  "<VINP_FlashAirIntenZone3MSet5_enum>"
  Bus Selector/42 -> ThermalControl/177(EEP_AirIntenZone3MSet7)  "<VINP_FlashAirIntenZone3MSet7_enum>"
  Bus Selector/43 -> ThermalControl/178(EEP_FDCFGSChStaSet457)  "<VINP_FlashFGSChStaSet457_enum>"
  Bus Selector/44 -> ThermalControl/179(EEP_FDCFGSAirIntStaSet457)  "<VINP_FlashFGSAirIntStaSet457_enum>"
  Bus Selector/45 -> ThermalControl/180(EEP_FDCTHCLEVentModeStaSet457)  "<VINP_FlashLEVentModeStaSet457_enum>"
  Bus Selector/46 -> ThermalControl/181(EEP_FDCTHCREVentModeStaSet457)  "<VINP_FlashREVentModeStaSet457_enum>"
  Bus Selector/47 -> ThermalControl/182(EEP_FDCTHCLEVentZStaSet2)  "<VINP_FlashLEVentZStaSet2_enum>"
  Bus Selector/48 -> ThermalControl/183(EEP_FDCTHCLEVentZStaSet3)  "<VINP_FlashLEVentZStaSet3_enum>"
  Bus Selector/49 -> ThermalControl/184(EEP_FDCTHCLEVentZStaSet4)  "<VINP_FlashLEVentZStaSet4_enum>"
  Bus Selector/50 -> ThermalControl/185(EEP_FDCTHCLEVentZStaSet5)  "<VINP_FlashLEVentZStaSet5_enum>"
  Bus Selector/51 -> ThermalControl/186(EEP_FDCTHCLEVentZStaSet7)  "<VINP_FlashLEVentZStaSet7_enum>"
  Bus Selector/52 -> ThermalControl/187(EEP_FDCTHCCLEVentZStaSet2)  "<VINP_FlashCLEVentZStaSet2_enum>"
  Bus Selector/53 -> ThermalControl/188(EEP_FDCTHCCLEVentZStaSet3)  "<VINP_FlashCLEVentZStaSet3_enum>"
  Bus Selector/54 -> ThermalControl/189(EEP_FDCTHCCLEVentZStaSet4)  "<VINP_FlashCLEVentZStaSet4_enum>"
  Bus Selector/55 -> ThermalControl/190(EEP_FDCTHCCLEVentZStaSet5)  "<VINP_FlashCLEVentZStaSet5_enum>"
  Bus Selector/56 -> ThermalControl/191(EEP_FDCTHCCLEVentZStaSet7)  "<VINP_FlashCLEVentZStaSet7_enum>"
  Bus Selector/57 -> ThermalControl/192(EEP_FDCTHCREVentZStaSet2)  "<VINP_FlashREVentZStaSet2_enum>"
  Bus Selector/58 -> ThermalControl/193(EEP_FDCTHCREVentZStaSet3)  "<VINP_FlashREVentZStaSet3_enum>"
  Bus Selector/59 -> ThermalControl/194(EEP_FDCTHCREVentZStaSet4)  "<VINP_FlashREVentZStaSet4_enum>"
  Bus Selector/60 -> ThermalControl/195(EEP_FDCTHCREVentZStaSet5)  "<VINP_FlashREVentZStaSet5_enum>"
  Bus Selector/61 -> ThermalControl/196(EEP_FDCTHCREVentZStaSet7)  "<VINP_FlashREVentZStaSet7_enum>"
  Bus Selector/62 -> ThermalControl/197(EEP_FDCTHCCREVentZStaSet2)  "<VINP_FlashCREVentZStaSet2_enum>"
  Bus Selector/63 -> ThermalControl/198(EEP_FDCTHCCREVentZStaSet3)  "<VINP_FlashCREVentZStaSet3_enum>"
  Bus Selector/64 -> ThermalControl/199(EEP_FDCTHCCREVentZStaSet4)  "<VINP_FlashCREVentZStaSet4_enum>"
  Bus Selector/65 -> ThermalControl/200(EEP_FDCTHCCREVentZStaSet5)  "<VINP_FlashCREVentZStaSet5_enum>"
  Bus Selector/66 -> ThermalControl/201(EEP_FDCTHCCREVentZStaSet7)  "<VINP_FlashCREVentZStaSet7_enum>"
  Bus Selector/67 -> ThermalControl/202(EEP_FDCTHCLEVentYStaSet2)  "<VINP_FlashLEVentYStaSet2_enum>"
  Bus Selector/68 -> ThermalControl/203(EEP_FDCTHCLEVentYStaSet3)  "<VINP_FlashLEVentYStaSet3_enum>"
  Bus Selector/69 -> ThermalControl/204(EEP_FDCTHCLEVentYStaSet4)  "<VINP_FlashLEVentYStaSet4_enum>"
  Bus Selector/70 -> ThermalControl/205(EEP_FDCTHCLEVentYStaSet5)  "<VINP_FlashLEVentYStaSet5_enum>"
  Bus Selector/71 -> ThermalControl/206(EEP_FDCTHCLEVentYStaSet7)  "<VINP_FlashLEVentYStaSet7_enum>"
  Bus Selector/72 -> ThermalControl/207(EEP_FDCTHCCLEVentYStaSet2)  "<VINP_FlashCLEVentYStaSet2_enum>"
  Bus Selector/73 -> ThermalControl/208(EEP_FDCTHCCLEVentYStaSet3)  "<VINP_FlashCLEVentYStaSet3_enum>"
  Bus Selector/74 -> ThermalControl/209(EEP_FDCTHCCLEVentYStaSet4)  "<VINP_FlashCLEVentYStaSet4_enum>"
  Bus Selector/75 -> ThermalControl/210(EEP_FDCTHCCLEVentYStaSet5)  "<VINP_FlashCLEVentYStaSet5_enum>"
  Bus Selector/76 -> ThermalControl/211(EEP_FDCTHCCLEVentYStaSet7)  "<VINP_FlashCLEVentYStaSet7_enum>"
  Bus Selector/77 -> ThermalControl/212(EEP_FDCTHCREVentYStaSet2)  "<VINP_FlashREVentYStaSet2_enum>"
  Bus Selector/78 -> ThermalControl/213(EEP_FDCTHCREVentYStaSet3)  "<VINP_FlashREVentYStaSet3_enum>"
  Bus Selector/79 -> ThermalControl/214(EEP_FDCTHCREVentYStaSet4)  "<VINP_FlashREVentYStaSet4_enum>"
  Bus Selector/80 -> ThermalControl/215(EEP_FDCTHCREVentYStaSet5)  "<VINP_FlashREVentYStaSet5_enum>"
  Bus Selector/81 -> ThermalControl/216(EEP_FDCTHCREVentYStaSet7)  "<VINP_FlashREVentYStaSet7_enum>"
  Bus Selector/82 -> ThermalControl/217(EEP_FDCTHCCREVentYStaSet2)  "<VINP_FlashCREVentYStaSet2_enum>"
  Bus Selector/83 -> ThermalControl/218(EEP_FDCTHCCREVentYStaSet3)  "<VINP_FlashCREVentYStaSet3_enum>"
  Bus Selector/84 -> ThermalControl/219(EEP_FDCTHCCREVentYStaSet4)  "<VINP_FlashCREVentYStaSet4_enum>"
  Bus Selector/85 -> ThermalControl/220(EEP_FDCTHCCREVentYStaSet5)  "<VINP_FlashCREVentYStaSet5_enum>"
  Bus Selector/86 -> ThermalControl/221(EEP_FDCTHCCREVentYStaSet7)  "<VINP_FlashCREVentYStaSet7_enum>"
  Bus Selector/87 -> ThermalControl/222(EEP_ACModeSet457)  "<VINP_FlashACModeSet457_enum>"
  Bus Selector/88 -> ThermalControl/223(EEP_SettempZon1Set2)  "<VINP_FlashSettempZon1Set2_enum>"
  Bus Selector/89 -> ThermalControl/224(EEP_SettempZon1Set3)  "<VINP_FlashSettempZon1Set3_enum>"
  Bus Selector/90 -> ThermalControl/225(EEP_SettempZon1Set4)  "<VINP_FlashSettempZon1Set4_enum>"
  Bus Selector/91 -> ThermalControl/226(EEP_SettempZon1Set5)  "<VINP_FlashSettempZon1Set5_enum>"
  Bus Selector/92 -> ThermalControl/227(EEP_SettempZon1Set7)  "<VINP_FlashSettempZon1Set7_enum>"
  ThermalControl/196(VTHC_LVentEN_flg) -> Bus Creator/196
  ThermalControl/197(VTHC_CLVentEN_flg) -> Bus Creator/197
  ThermalControl/198(VTHC_RVentEN_flg) -> Bus Creator/198
  ThermalControl/199(VTHC_CRVentEN_flg) -> Bus Creator/199
  ThermalControl/200(VTHC_FDCFGSLearnCmd_enum) -> Bus Creator/200
  Bus Selector/13 -> ThermalControl/148(EEP_SettempZon1Set1)  "<VINP_FlashsigSetTempZon1St_C>"
  ThermalControl/201(VTHC_FDCFGSFuncSta_flg) -> Bus Creator/201
  BINP_CAN5_outputs/1 -> Terminator/1
  BINP_SYS_outputs/1 -> [BINP_SYS_outputs]  "BINP_SYS_output"
  [BINP_SYS_outputs] -> Bus Selector/1
  [BINP_SYS_outputs] -> Bus Selector6/1
  Bus Selector7/2 -> ThermalControl/2(VPMM_SysPwrSta_enum)  "<VPMM_SysPowerMode_enum>"
  ThermalControl/202(VTHC_THSysErrlampReq_flg) -> Bus Creator/202
